simulink model "converter_2021b"  (R2021b)
settings: Solver=FixedStepAuto  StartTime=0.0  StopTime=10.0  FixedStep=SIM.Ts  MaxStep=SIM.Ts  RelTol=1e-3
values from neighbouring files (symbols this model uses):
  Ts = SIM.Ts    [RUN_Loss_Tool.m]
undefined symbols (not defined in the file or in its folder): plecs
libraries: LossSim_Library x8
settings Model: Creator=Milan Utvic  LastModifiedBy=baliu
settings SolverCC: InitialStep=SIM.Ts/2  AlgebraicLoopSolver=TrustRegion
settings DataIOCC: SaveFormat=StructureWithTime  ReturnWorkspaceOutputs=off
settings OptimizationCC: LifeSpan=inf
settings DebuggingCC: SFExecutionAtInitializationDiag=none  ArithmeticOperatorsInVariantConditions=warning
settings HardwareCC: ProdBitPerSizeT=32  ProdBitPerPtrDiffT=32  ProdWordSize=32  ProdHWDeviceType=Specified
settings SFSimCC: SimUseLocalCustomCode=off  CustomCodeUndefinedFunction=UseInterfaceOnly
settings RTWCC: RTWUseLocalCustomCode=off
settings CodeAppCC: StateflowObjectComments=on
settings ConfigComp: CovBoundaryAbsTol=1.0e-5

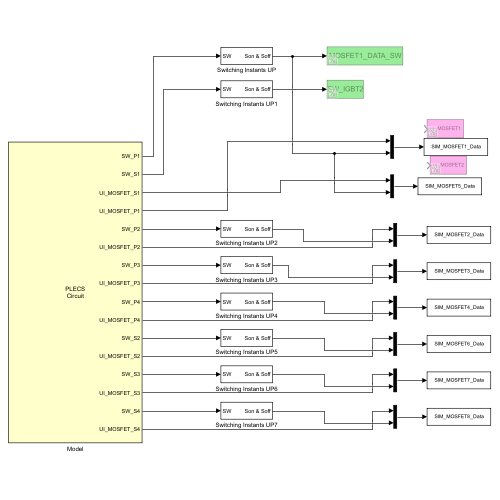
[thumbnail: Simulink's stored preview of the top-level diagram]
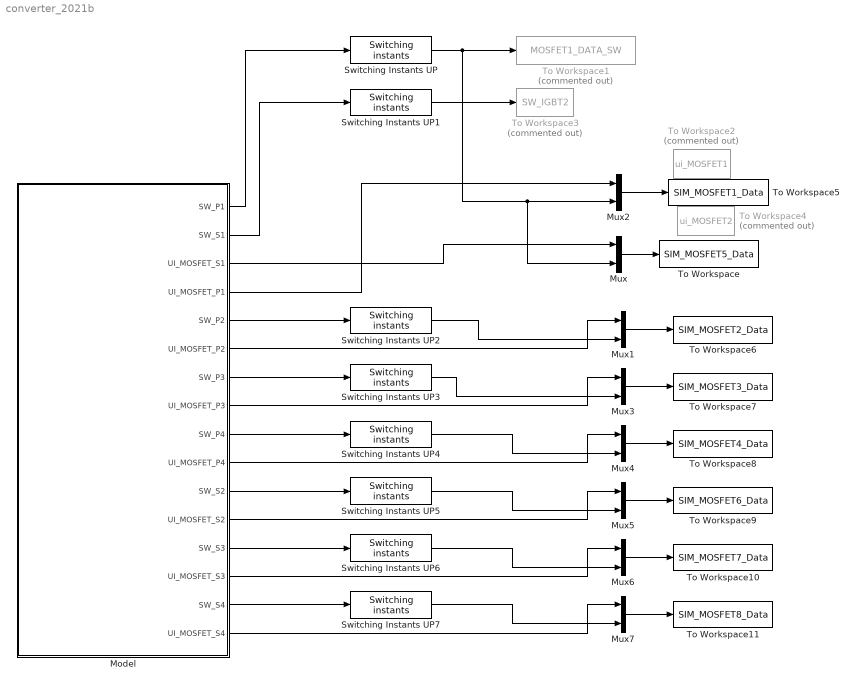
== system converter_2021b ==
  Model : Subsystem  LoadFcn=plecs('sl', 200);  InitFcn=plecs('sl', 214);  StartFcn=plecs('sl', 208);  StopFcn=plecs('sl', 209);  ClipboardFcn=plecs('sl', 212, 12);  mask(PlecsCircuit){PLECSData=<binary blob, 9492 chars, not shown>}
      mask prompts: PLECSData "PLECS Data (Do not delete or modify!)"
      mask init:
      | % PLACE CUSTOM INITIALIZATIONS ABOVE
      | % DO NOT REMOVE
      | plecs('sl', 215);
      | % DO NOT REMOVE
      settings: CopyFcn=plecs('sl', 203);  DeleteFcn=plecs('sl', 205);  UndoDeleteFcn=plecs('sl', 206);  PreSaveFcn=plecs('sl', 211);  PostSaveFcn=plecs('sl', 201);  NameChangeFcn=plecs('sl', 210);  DestroyFcn=plecs('sl', 207);  PreCopyFcn=plecs('sl', 216);  OpenFcn=plecs('sl', 202);  ErrorFcn=plerrorfcn
      mask Help: web(['file:///' fullfile(plecsdoc, 'creatingacircuit.html')])
      mask Display: disp('PLECS\nCircuit')
  Mux{,1..7} (8 alike) : Mux  Inputs=2
  Switching Instants UP{,1..7} (8 alike) : LossSim_Library/Switching instants  SystemSampleTime=-1  VariantActivationTime=update diagram  EmptyChoice=off  PassThrough=off  PassThroughVariantControl=(default)  EmptyChoiceVariantControl=(default)  Latency=0  AutoFrameSizeCalculation=off
  To Workspace : ToWorkspace  VariableName=SIM_MOSFET5_Data  SampleTime=Ts
      settings: MaxDataPoints=NOS
  To Workspace1 : ToWorkspace  Commented=on  VariableName=MOSFET1_DATA_SW  SampleTime=Ts
      settings: MaxDataPoints=NOS
  To Workspace10 : ToWorkspace  VariableName=SIM_MOSFET7_Data  SampleTime=Ts
      settings: MaxDataPoints=NOS
  To Workspace11 : ToWorkspace  VariableName=SIM_MOSFET8_Data  SampleTime=Ts
      settings: MaxDataPoints=NOS
  To Workspace2 : ToWorkspace  Commented=on  VariableName=ui_MOSFET1  SampleTime=Ts
      settings: MaxDataPoints=NOS
  To Workspace3 : ToWorkspace  Commented=on  VariableName=SW_IGBT2  SampleTime=Ts
      settings: MaxDataPoints=NOS
  To Workspace4 : ToWorkspace  Commented=on  VariableName=ui_MOSFET2  SampleTime=Ts
      settings: MaxDataPoints=NOS
  To Workspace5 : ToWorkspace  VariableName=SIM_MOSFET1_Data  SampleTime=Ts
      settings: MaxDataPoints=NOS
  To Workspace6 : ToWorkspace  VariableName=SIM_MOSFET2_Data  SampleTime=Ts
      settings: MaxDataPoints=NOS
  To Workspace7 : ToWorkspace  VariableName=SIM_MOSFET3_Data  SampleTime=Ts
      settings: MaxDataPoints=NOS
  To Workspace8 : ToWorkspace  VariableName=SIM_MOSFET4_Data  SampleTime=Ts
      settings: MaxDataPoints=NOS
  To Workspace9 : ToWorkspace  VariableName=SIM_MOSFET6_Data  SampleTime=Ts
      settings: MaxDataPoints=NOS
  wires:
  Switching Instants UP/1 -> To Workspace1/1, Mux/2, Mux2/2
  Mux/1 -> To Workspace/1
  Switching Instants UP1/1 -> To Workspace3/1
  Model/1(SW_P1) -> Switching Instants UP/1
  Model/2(SW_S1) -> Switching Instants UP1/1
  Mux2/1 -> To Workspace5/1
  Model/4(UI_MOSFET_P1) -> Mux2/1
  Model/3(UI_MOSFET_S1) -> Mux/1
  Model/5(SW_P2) -> Switching Instants UP2/1
  Model/6(UI_MOSFET_P2) -> Mux1/1
  Mux1/1 -> To Workspace6/1
  Model/7(SW_P3) -> Switching Instants UP3/1
  Model/8(UI_MOSFET_P3) -> Mux3/1
  Mux3/1 -> To Workspace7/1
  Model/9(SW_P4) -> Switching Instants UP4/1
  Model/10(UI_MOSFET_P4) -> Mux4/1
  Mux4/1 -> To Workspace8/1
  Model/11(SW_S2) -> Switching Instants UP5/1
  Model/12(UI_MOSFET_S2) -> Mux5/1
  Mux5/1 -> To Workspace9/1
  Model/13(SW_S3) -> Switching Instants UP6/1
  Model/14(UI_MOSFET_S3) -> Mux6/1
  Mux6/1 -> To Workspace10/1
  Model/15(SW_S4) -> Switching Instants UP7/1
  Model/16(UI_MOSFET_S4) -> Mux7/1
  Mux7/1 -> To Workspace11/1
  Switching Instants UP2/1 -> Mux1/2
  Switching Instants UP3/1 -> Mux3/2
  Switching Instants UP4/1 -> Mux4/2
  Switching Instants UP5/1 -> Mux5/2
  Switching Instants UP6/1 -> Mux6/2
  Switching Instants UP7/1 -> Mux7/2

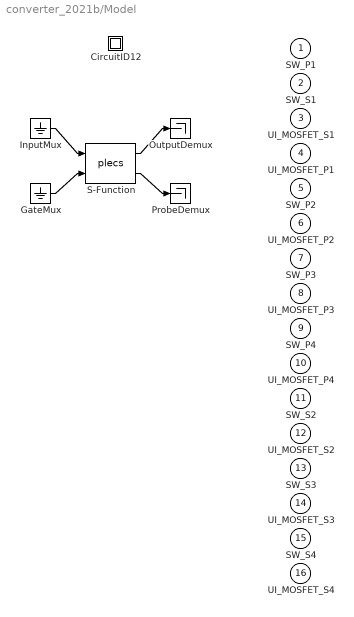
== system converter_2021b/Model ==
  " CircuitID12 " : Subsystem
  " GateMux " : Ground
  " InputMux " : Ground
  " OutputDemux " : Terminator
  " ProbeDemux " : Terminator
  " S-Function " : S-Function  FunctionName=plecs  SFunctionDeploymentMode=off  EnableBusSupport=off
  SW_P1 : Outport  PortDimensions=1
  SW_S1 : Outport  Port=2  PortDimensions=1
  UI_MOSFET_S1 : Outport  Port=3  PortDimensions=2
  UI_MOSFET_P1 : Outport  Port=4  PortDimensions=2
  SW_P2 : Outport  Port=5  PortDimensions=1
  UI_MOSFET_P2 : Outport  Port=6  PortDimensions=2
  SW_P3 : Outport  Port=7  PortDimensions=1
  UI_MOSFET_P3 : Outport  Port=8  PortDimensions=2
  SW_P4 : Outport  Port=9  PortDimensions=1
  UI_MOSFET_P4 : Outport  Port=10  PortDimensions=2
  SW_S2 : Outport  Port=11  PortDimensions=1
  UI_MOSFET_S2 : Outport  Port=12  PortDimensions=2
  SW_S3 : Outport  Port=13  PortDimensions=1
  UI_MOSFET_S3 : Outport  Port=14  PortDimensions=2
  SW_S4 : Outport  Port=15  PortDimensions=1
  UI_MOSFET_S4 : Outport  Port=16  PortDimensions=2
  wires:
  " InputMux "/1 -> " S-Function "/1
  " GateMux "/1 -> " S-Function "/2
  " S-Function "/1 -> " OutputDemux "/1
  " S-Function "/2 -> " ProbeDemux "/1

== system converter_2021b/Model/ CircuitID12  ==
